simulink model "CSEI_model"  (R2015b)
settings: Solver=VariableStepAuto  StartTime=0.0  StopTime=5000  RelTol=1e-3
values from neighbouring files (symbols this model uses):
  b = [0;0;0]    [script_backstepping.m]
  D = [-X_u,0,0 ... (first row only)    [script_backstepping.m]
  eta0 = [p0(1);p0(2);psi0]    [script_backstepping.m]
  integrator_reset = 0    [script_backstepping.m]
  K1 = diag([0.1, 0.2 ,0.1])    [script_backstepping.m]
  K2 = diag([0.1, 0.2, 0.1])    [script_backstepping.m]
  M = [m-X_u_dot,0,0 ... (first row only)    [script_backstepping.m]
  mu = 10    [script.m]    (also in script_backstepping.m = 2)
  pd_0 = [2;0]    [script.m]    (also in script_backstepping.m)
  pd_1 = [10;4]    [script.m]    (also in script_backstepping.m)
  U_max = 0.4    [script.m]    (also in script_backstepping.m = 0.1)
settings Model: Creator=Shiv Jeet rai  LastModifiedBy=Shiv Jeet rai

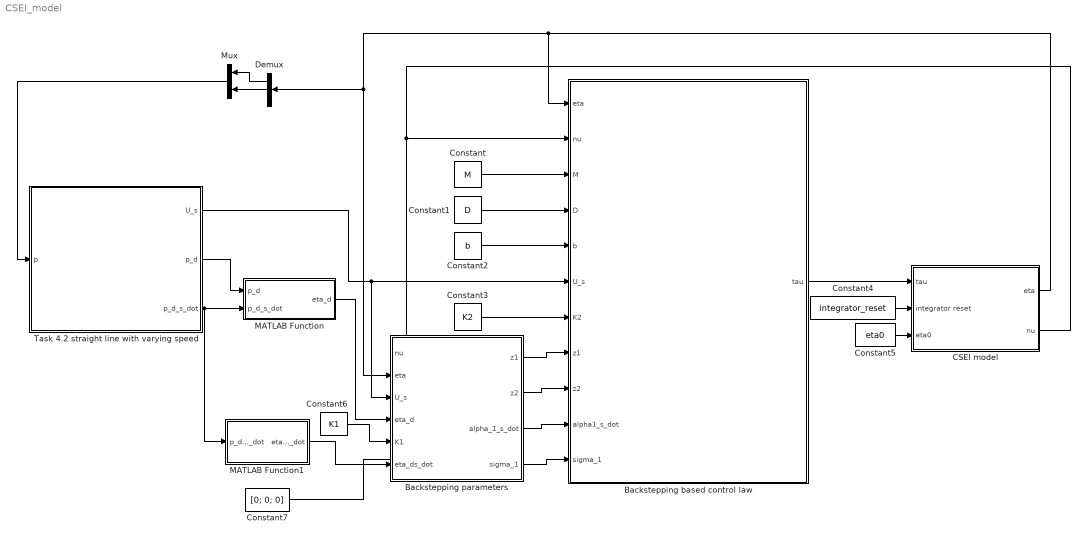
== system CSEI_model ==
  Backstepping based control law : MATLAB Function  TreatAsAtomicUnit=on
  Backstepping parameters : Subsystem
  CSEI model : Subsystem
  Constant : Constant  Value=M
  Constant1 : Constant  Value=D
  Constant2 : Constant  Value=b
  Constant3 : Constant  Value=K2
  Constant4 : Constant  Value=integrator_reset
  Constant5 : Constant  Value=eta0
  Constant6 : Constant  Value=K1
  Constant7 : Constant  Value=[0; 0; 0]
  Demux : Demux  Outputs=3
  MATLAB Function : MATLAB Function  TreatAsAtomicUnit=on
  MATLAB Function1 : MATLAB Function  TreatAsAtomicUnit=on
  Mux : Mux  Inputs=2
  Task 4.2 straight line with varying speed : Subsystem
  wires:
  Backstepping based control law/1(tau) -> CSEI model/1(tau)
  Backstepping parameters/1(z1) -> Backstepping based control law/8(z1)
  Backstepping parameters/2(z2) -> Backstepping based control law/9(z2)
  Backstepping parameters/3(alpha_1_s_dot) -> Backstepping based control law/10(alpha1_s_dot)
  Backstepping parameters/4(sigma_1) -> Backstepping based control law/11(sigma_1)
  CSEI model/2(nu) -> Backstepping parameters/1("nu "), Backstepping based control law/2(nu)
  Constant/1 -> Backstepping based control law/3(M)
  Constant1/1 -> Backstepping based control law/4(D)
  Constant2/1 -> Backstepping based control law/5(b)
  Constant3/1 -> Backstepping based control law/7(K2)
  Task 4.2 straight line with varying speed/1(U_s) -> Backstepping parameters/3(U_s), Backstepping based control law/6(U_s)
  Constant4/1 -> CSEI model/2(integrator reset)
  Constant5/1 -> CSEI model/3(eta0)
  Constant6/1 -> Backstepping parameters/5(K1)
  MATLAB Function/1(eta_d) -> Backstepping parameters/4(eta_d)
  MATLAB Function1/1(eta_ds_dot) -> Backstepping parameters/6(eta_ds_dot)
  Constant7/1 -> ?
  Task 4.2 straight line with varying speed/3(p_d_s_dot) -> MATLAB Function1/1(p_d_s_dot), MATLAB Function/2(p_d_s_dot)
  Task 4.2 straight line with varying speed/2(p_d) -> MATLAB Function/1(p_d)
  Mux/1 -> Task 4.2 straight line with varying speed/1(p)
  CSEI model/1(eta) -> Backstepping based control law/1(eta), Demux/1, Backstepping parameters/2(eta)
  Demux/1 -> Mux/1
  Demux/2 -> Mux/2

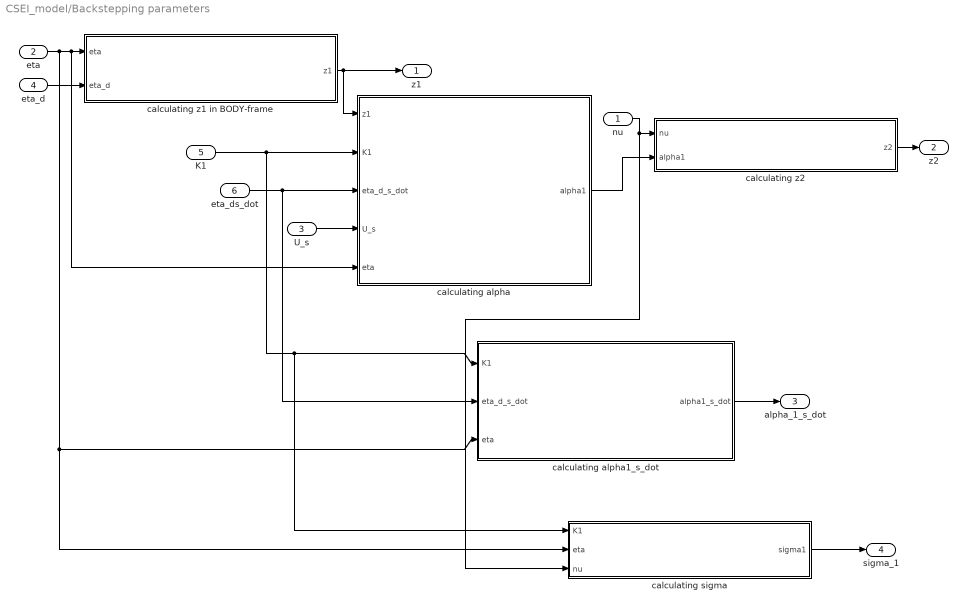
== system CSEI_model/Backstepping parameters ==
  "nu " : Inport
  eta : Inport  Port=2
  U_s : Inport  Port=3
  eta_d : Inport  Port=4
  K1 : Inport  Port=5
  eta_ds_dot : Inport  Port=6
  calculating alpha : MATLAB Function  TreatAsAtomicUnit=on
  calculating alpha1_s_dot : MATLAB Function  TreatAsAtomicUnit=on
  "calculating sigma " : MATLAB Function  TreatAsAtomicUnit=on
  calculating z1 in BODY-frame : MATLAB Function  TreatAsAtomicUnit=on
  calculating z2 : MATLAB Function  TreatAsAtomicUnit=on
  z1 : Outport
  z2 : Outport  Port=2
  alpha_1_s_dot : Outport  Port=3
  sigma_1 : Outport  Port=4
  wires:
  calculating z1 in BODY-frame/1(z1) -> calculating alpha/1(z1), z1/1
  calculating z2/1(z2) -> z2/1
  "nu "/1 -> "calculating sigma "/3(nu), calculating z2/1(nu)
  eta_d/1 -> calculating z1 in BODY-frame/2(eta_d)
  calculating alpha/1(alpha1) -> calculating z2/2(alpha1)
  eta_ds_dot/1 -> calculating alpha1_s_dot/2(eta_d_s_dot), calculating alpha/3(eta_d_s_dot)
  U_s/1 -> calculating alpha/4(U_s)
  calculating alpha1_s_dot/1(alpha1_s_dot) -> alpha_1_s_dot/1
  "calculating sigma "/1(sigma1) -> sigma_1/1
  K1/1 -> "calculating sigma "/1(K1), calculating alpha1_s_dot/1(K1), calculating alpha/2(K1)
  eta/1 -> "calculating sigma "/2(eta), calculating alpha1_s_dot/3(eta), calculating alpha/5(eta), calculating z1 in BODY-frame/1(eta)

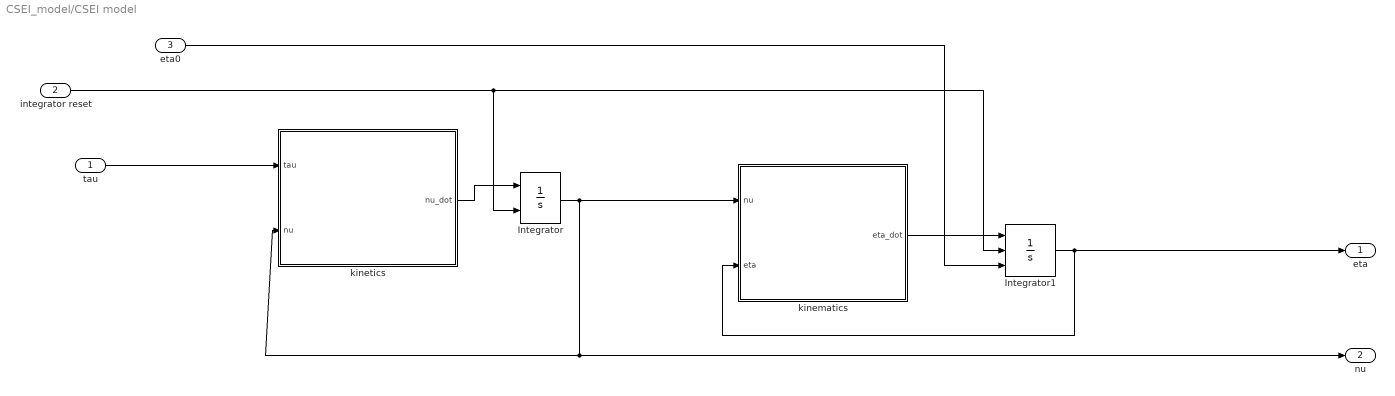
== system CSEI_model/CSEI model ==
  tau : Inport
  integrator reset : Inport  Port=2
  eta0 : Inport  Port=3
  Integrator : Integrator  ExternalReset=rising  InitialCondition=[0 0 0]'
  Integrator1 : Integrator  ExternalReset=rising  InitialConditionSource=external  InitialCondition=[0 0 0]'
  kinematics : MATLAB Function  TreatAsAtomicUnit=on
  kinetics : MATLAB Function  TreatAsAtomicUnit=on
  eta : Outport
  nu : Outport  Port=2
  wires:
  kinematics/1(eta_dot) -> Integrator1/1
  Integrator/1 -> nu/1, kinetics/2(nu), kinematics/1(nu)
  eta0/1 -> Integrator1/3
  kinetics/1(nu_dot) -> Integrator/1
  Integrator1/1 -> eta/1, kinematics/2(eta)
  tau/1 -> kinetics/1(tau)
  integrator reset/1 -> Integrator1/2, Integrator/2

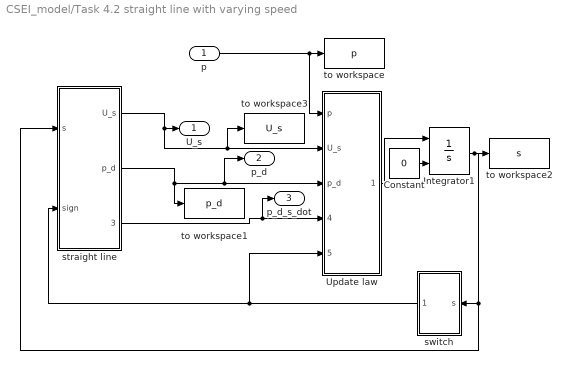
== system CSEI_model/Task 4.2 straight line with varying speed ==
  p : Inport
  Constant : Constant  Value=0
  Integrator1 : Integrator  InitialConditionSource=external
  Update law : Subsystem
  straight line : Subsystem
  switch : Subsystem
  to workspace : ToWorkspace  VariableName=p  SaveFormat=Timeseries  SampleTime=-1
  to workspace1 : ToWorkspace  VariableName=p_d  SaveFormat=Timeseries  SampleTime=-1
  to workspace2 : ToWorkspace  VariableName=s  SaveFormat=Timeseries  SampleTime=-1
  to workspace3 : ToWorkspace  VariableName=U_s  SaveFormat=Timeseries  SampleTime=-1
  U_s : Outport
  p_d : Outport  Port=2
  p_d_s_dot : Outport  Port=3
  wires:
  Update law/1(s_dot) -> Integrator1/1
  switch/1(sign) -> Update law/5(sigma), straight line/2(sign)
  straight line/3(p_d_s_dot) -> p_d_s_dot/1, Update law/4(p_d_s_dot)
  Constant/1 -> Integrator1/2
  straight line/2(p_d) -> to workspace1/1, p_d/1, Update law/3(p_d)
  straight line/1(U_s) -> to workspace3/1, Update law/2(U_s), U_s/1
  Integrator1/1 -> straight line/1(s), switch/1(s), to workspace2/1
  p/1 -> Update law/1(p), to workspace/1

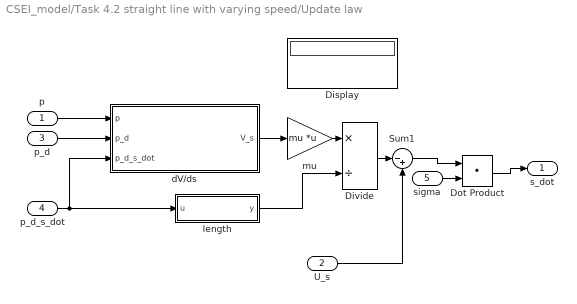
== system CSEI_model/Task 4.2 straight line with varying speed/Update law ==
  p : Inport
  U_s : Inport  Port=2
  p_d : Inport  Port=3
  p_d_s_dot : Inport  Port=4
  sigma : Inport  Port=5
  Display : Display
  Divide : Product  Inputs=*/
  Dot Product : DotProduct  InputSameDT=on  OutDataTypeStr=Inherit: Inherit via internal rule
  Sum1 : Sum  Inputs=|-+
  "dV/ds  " : MATLAB Function  TreatAsAtomicUnit=on
  length : MATLAB Function  TreatAsAtomicUnit=on
  mu : Gain  Gain=mu  Multiplication=Matrix(K*u)
  s_dot : Outport
  wires:
  p/1 -> "dV/ds  "/1(p)
  mu/1 -> Divide/1
  Divide/1 -> Sum1/1
  "dV/ds  "/1(V_s) -> mu/1
  p_d/1 -> "dV/ds  "/2(p_d)
  p_d_s_dot/1 -> "dV/ds  "/3(p_d_s_dot), length/1(u)
  length/1(y) -> Divide/2
  U_s/1 -> Sum1/2
  Sum1/1 -> Dot Product/1
  Dot Product/1 -> s_dot/1
  sigma/1 -> Dot Product/2

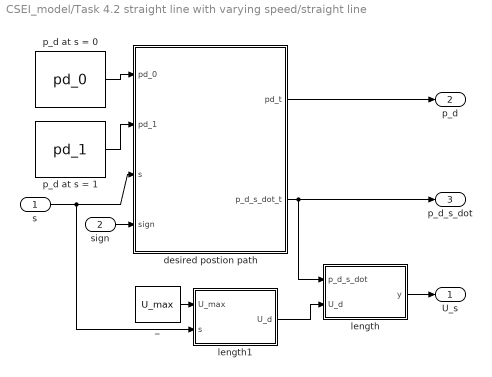
== system CSEI_model/Task 4.2 straight line with varying speed/straight line ==
  s : Inport
  sign : Inport  Port=2
  _ : Constant  Value=U_max
  desired postion path : MATLAB Function  TreatAsAtomicUnit=on
  length : MATLAB Function  TreatAsAtomicUnit=on
  length1 : MATLAB Function  TreatAsAtomicUnit=on
  p_d at s = 0 : Constant  Value=pd_0
  p_d at s = 1 : Constant  Value=pd_1
  U_s : Outport
  p_d : Outport  Port=2
  p_d_s_dot : Outport  Port=3
  wires:
  p_d at s = 1/1 -> desired postion path/2(pd_1)
  p_d at s = 0/1 -> desired postion path/1(pd_0)
  desired postion path/1(pd_t) -> p_d/1
  desired postion path/2(p_d_s_dot_t) -> length/1(p_d_s_dot), p_d_s_dot/1
  length/1(y) -> U_s/1
  s/1 -> length1/2(s), desired postion path/3(s)
  sign/1 -> desired postion path/4(sign)
  _/1 -> length1/1(U_max)
  length1/1(U_d) -> length/2(U_d)

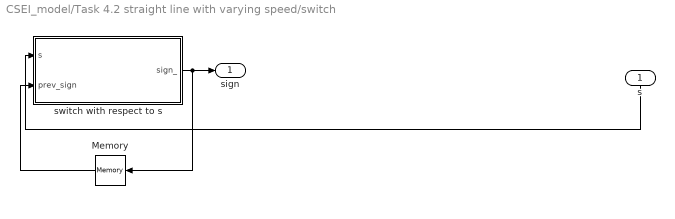
== system CSEI_model/Task 4.2 straight line with varying speed/switch ==
  s : Inport
  Memory : Memory  X0=1
  switch with respect to s : MATLAB Function  TreatAsAtomicUnit=on
  sign : Outport
  wires:
  switch with respect to s/1(sign_) -> sign/1, Memory/1
  Memory/1 -> switch with respect to s/2(prev_sign)
  s/1 -> switch with respect to s/1(s)

== matlab function CSEI_model/CSEI model/kinematics ==
  data: nu input; eta_dot output; eta input
function eta_dot = CSE1_eta_dot(nu,eta)

psi = eta(3);

J = [cos(psi) -sin(psi) 0
     sin(psi) cos(psi)  0
     0        0         1];

eta_dot = J*nu;

== matlab function CSEI_model/CSEI model/kinetics ==
  data: tau input; nu_dot output; nu input
function nu_dot = CSE1_nu_dot(tau,nu)

u   = nu(1);
v   = nu(2);
r   = nu(3);

tau = [tau(1);tau(2);tau(3)];
%% MATRICES

m    = 14.79;   I_z  =  1.7600;   x_g = 0.0375;       % x_g  =  0.0460; % Table B.1


%% Added mass
X_ud  =     -2.0;											% Table B.1
					Y_vd =     -1.0;	N_vd =    -0.0;		% Table B.1 guestimate
					Y_rd =      -0.0;	N_rd =    -1.0;		% Table B.1

%% Total mass matrix
m_11 = m-X_ud;
m_22 = m-Y_vd;
m_23 = m*x_g-Y_rd;
m_32 = m*x_g-N_vd;
m_33 = I_z-N_rd;

M    = [m_11 0    0
        0    m_22 m_23
        0    m_32 m_33];
	
%% Damping coefficients
% Comments at the end of the lines indicate the old values used.
X_u		= -0.6555;		X_v		= 0;
X_uu 	= 0.3545;		X_vv	= -2.443;
X_uuu 	= -3.787;		X_vvv	= 0;

						Y_v		= -1.33; 			Y_r		= -7.250; % Y_r
						Y_vv	= -2.776;			Y_rr	= -3.450; % Y_rr
						Y_vvv	= -64.91;			Y_rrr	= 0;
						
						Y_rv	= -0.805;			Y_vr	= -0.845; % Y_rv, Y_vr

						N_v		= 0;				N_r		= -1.900; % N_r
						N_vv	= -0.2088;			N_rr	= -0.750; % N_rr
						N_vvv	= 0;				N_rrr	= 0;
						
						N_rv	= 0.130;			N_vr	= 0.080; % N_rv, N_vr

%% Correolis matrix
c_13 = -(m-Y_vd)*v-(m*x_g-Y_rd)*r;
c_23 = (m-X_ud)*u;
C    = [0     0     c_13
        0     0     c_23
        -c_13 -c_23 0   ];

%% Assembly of the damping matrix
d_11 = -X_u - X_uu*u - X_uuu*u^2;
d_22 = -Y_v - Y_vv*v - Y_vvv*v^2 - Y_rv*abs(r);
d_33 = -N_r - N_rr*abs(r) - N_rrr*r^2 - N_vr*abs(v); % using abs(r)

d_12 = -X_v - X_vv*v - X_vvv*v^2;
d_23 = -Y_r - Y_rr*abs(r) - Y_rrr*r^2 - Y_vr*abs(v);
d_32 = -N_v - N_vv*v - N_vvv*v^2 - N_rv*abs(r);

D    = [d_11 d_12 0
        0    d_22 d_23
        0    d_32 d_33];



%% CALCULATION
nu_dot = M\(tau-(C+D)*nu);

== matlab function CSEI_model/Backstepping based control law ==
  data: eta input; nu input; M input; D input; b input; U_s input; K2 input; z1 input; tau output; z2 input; alpha1_s_dot input; sigma_1 input size=[3 1]
function tau = fcn(eta, nu, M, D, b, U_s, K2, z1, z2, alpha1_s_dot,sigma_1)
%#codegen
psi = eta(3);
R = [   cos(psi)    -sin(psi)   0;
        sin(psi)    cos(psi)    0;
        0           0           0;];  
tau = -z1 + D*nu - transpose(R)*b + M*alpha1_s_dot*U_s + M*sigma_1 - K2*z2;

== matlab function CSEI_model/Task 4.2 straight line with varying speed/Update law/length ==
  data: u input; y output
function y = fcn(u)

y = sqrt(u(1)^2 + u(2)^2);

== matlab function CSEI_model/Task 4.2 straight line with varying speed/Update law/dV//ds   ==
  data: p input; V_s output; p_d input; p_d_s_dot input
function V_s = fcn(p, p_d, p_d_s_dot)

temp = - transpose(p - p_d)*p_d_s_dot;
V_s = temp;

== matlab function CSEI_model/Task 4.2 straight line with varying speed/straight line/length1 ==
  data: U_max input; U_d output; s input
function U_d = fcn(U_max,s)

if s > 1
    s = 1;
elseif s < 0
    s = 0;
end

U_d = U_max*(1.01 + sin(2*pi*s - pi/2))/2;

== matlab function CSEI_model/Backstepping parameters/calculating alpha ==
  data: z1 input size=[3 1]; K1 input; alpha1 output; eta_d_s_dot input size=[3 1]; U_s input size=1; eta input size=[3 1]
function alpha1 = fcn(z1,K1, eta_d_s_dot, U_s, eta)
%#codegen
psi = eta(3);
R = [   cos(psi)    -sin(psi)   0;
        sin(psi)    cos(psi)    0;
        0           0           0;];  

alpha1 = -K1*z1 + transpose(R)*eta_d_s_dot*U_s;

== matlab function CSEI_model/Task 4.2 straight line with varying speed/straight line/desired postion path ==
  data: pd_0 input; pd_1 input; pd_t output; p_d_s_dot_t output; s input size=1; sign input size=1
function [pd_t,p_d_s_dot_t] = fcn(pd_0,pd_1,s, sign)

if s >= 1,
    s = 1;
end

p_d_s_dot_t = [ (pd_1(1)-pd_0(1))*sign; 
                (pd_1(2)-pd_0(2))*sign];

pd_t =  [(pd_1(1)-pd_0(1))*s + pd_0(1);
         (pd_1(2)-pd_0(2))*s + pd_0(2)];   
end

== matlab function CSEI_model/Task 4.2 straight line with varying speed/straight line/length ==
  data: p_d_s_dot input; y output; U_d input
function y = fcn(p_d_s_dot,U_d)

y = U_d/sqrt(p_d_s_dot(1)^2 + p_d_s_dot(2)^2);

== matlab function CSEI_model/Backstepping parameters/calculating alpha1_s_dot ==
  data: K1 input size=[3 3]; eta_d_s_dot input size=[3 1]; alpha1_s_dot output size=[3 1]; eta input size=[3 1]
function alpha1_s_dot = fcn(K1, eta_d_s_dot, eta)
%#codegen
psi = eta(3);
R = [   cos(psi)    -sin(psi)   0;
        sin(psi)    cos(psi)    0;
        0           0           0;];  

alpha1_s_dot = K1*transpose(R)*eta_d_s_dot;

== matlab function CSEI_model/Backstepping parameters/calculating sigma  ==
  data: sigma1 output size=[3 1]; K1 input; eta input; nu input
function sigma1 = fcn(K1,eta,nu)
%Skew_symmetric_matrix =  
S = [0 -1 1;
     1 0 -1;
     -1 1 0;];

psi = eta(3);
R = [   cos(psi)    -sin(psi)   0;
        sin(psi)    cos(psi)    0;
        0           0           0;];

r = nu(3);
sigma1 = K1*S*eta*r - nu;

== matlab function CSEI_model/Backstepping parameters/calculating z1 in BODY-frame ==
  data: z1 output size=[3 1]; eta input size=[3 1]; eta_d input size=[3 1]
function z1 = fcn(eta, eta_d)
%#codegen
psi = eta(3);
R = [   cos(psi)    -sin(psi)   0;
        sin(psi)    cos(psi)    0;
        0           0           0;];  
z1 = transpose(R)*(eta-eta_d);

== matlab function CSEI_model/Backstepping parameters/calculating z2 ==
  data: z2 output size=[3 1]; nu input size=[3 1]; alpha1 input size=[3 1]
function z2 = fcn(nu, alpha1)
%#codegen

z2 = nu-alpha1;

== matlab function CSEI_model/Task 4.2 straight line with varying speed/switch/switch with respect to s ==
  data: s input; sign_ output; prev_sign input
function sign_ = fcn(s, prev_sign)

if s > 1 
    sign_ = -1;
elseif s <= 0
        sign_ = 1;
else
    sign_ = prev_sign;
end

== matlab function CSEI_model/MATLAB Function ==
  data: p_d input; p_d_s_dot input; eta_d output
function eta_d = fcn(p_d,p_d_s_dot)
%#codegen
psi_d = atan(p_d_s_dot(2)/p_d_s_dot(1));

eta_d = [p_d(1); p_d(2); psi_d];

== matlab function CSEI_model/MATLAB Function1 ==
  data: p_d_s_dot input; eta_ds_dot output
function eta_ds_dot = fcn(p_d_s_dot)
%#codegen
eta_ds_dot = [p_d_s_dot(1);p_d_s_dot(2);0];
